simulink model "Neurofeedback_StateSpace_Neurodynamics"  (R2021b)
settings: Solver=VariableStepAuto  StartTime=0.0  StopTime=300  FixedStep=0.1  RelTol=1e-3
settings Model: Creator=mdls3  LastModifiedBy=mariodelossantos

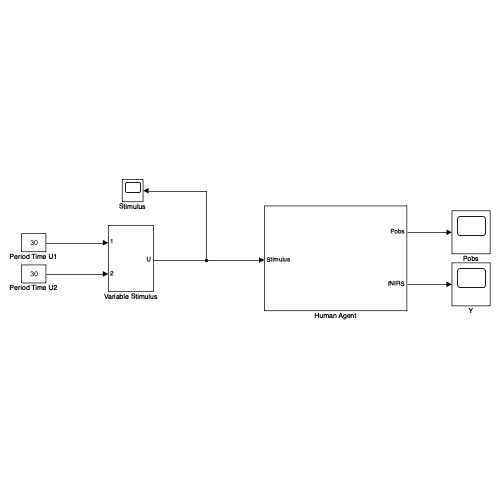
[thumbnail: Simulink's stored preview of the top-level diagram]
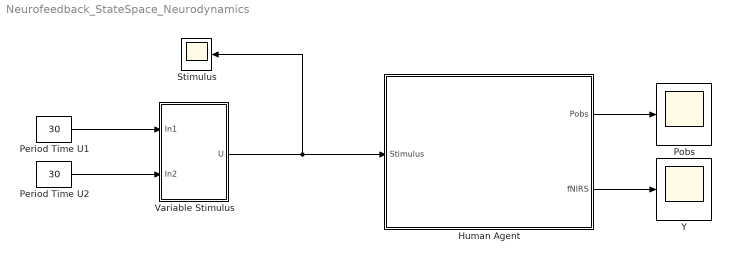
== system Neurofeedback_StateSpace_Neurodynamics ==
  Human Agent : Subsystem
  Period Time U1 : Constant  Value=30
  Period Time U2 : Constant  Value=30
  Pobs : Scope
  Stimulus : Scope
  Variable Stimulus : Subsystem
  Y : Scope
  wires:
  Period Time U1/1 -> Variable Stimulus/1(In1)
  Period Time U2/1 -> Variable Stimulus/2(In2)
  Variable Stimulus/1(U) -> Stimulus/1, Human Agent/1(Stimulus)
  Human Agent/2(fNIRS) -> Y/1
  Human Agent/1(Pobs) -> Pobs/1

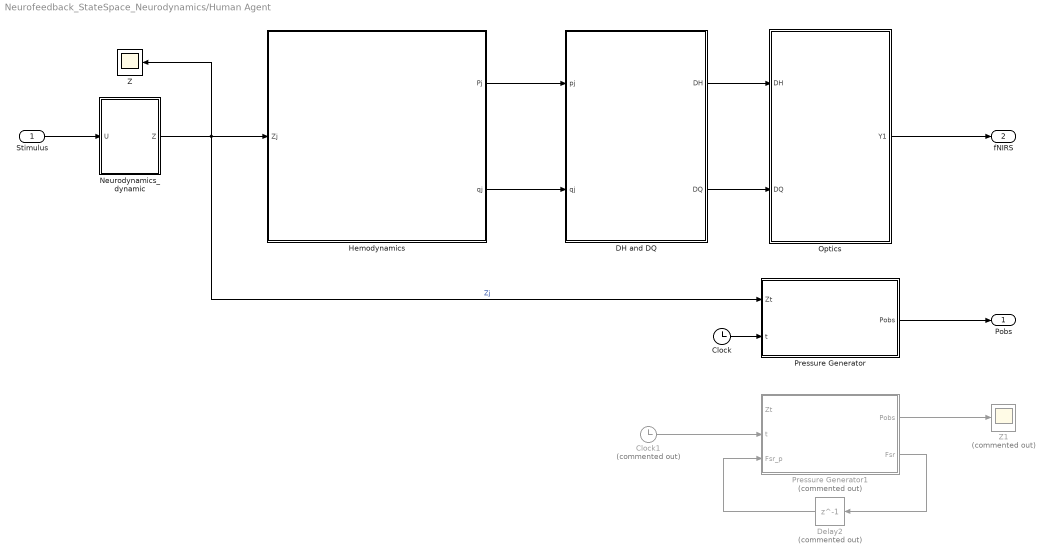
== system Neurofeedback_StateSpace_Neurodynamics/Human Agent ==
  Stimulus : Inport
  Clock : Clock
  Clock1 : Clock  Commented=on
  DH and DQ : Subsystem
  Delay2 : Delay  Commented=on  DelayLength=1  InitialCondition=0.0001
  Hemodynamics : Subsystem
  Neurodynamics_dynamic : Subsystem
  Optics : Subsystem
  Pressure Generator : MATLAB Function  TreatAsAtomicUnit=on
  Pressure Generator1 : MATLAB Function  Commented=on  TreatAsAtomicUnit=on
  Z : Scope
  Z1 : Scope  Commented=on
  Pobs : Outport
  fNIRS : Outport  Port=2
  wires:
  Hemodynamics/1(Pj) -> DH and DQ/1(pj)
  Hemodynamics/2(qj) -> DH and DQ/2(qj)
  Neurodynamics_dynamic/1(Z) -> Pressure Generator/1(Zt), Z/1, Hemodynamics/1(Zj)  "Zj"
  Stimulus/1 -> Neurodynamics_dynamic/1(U)
  DH and DQ/1(DH) -> Optics/1(DH)
  DH and DQ/2(DQ) -> Optics/2(DQ)
  Optics/1(Y1) -> fNIRS/1
  Clock/1 -> Pressure Generator/2(t)
  Pressure Generator/1(Pobs) -> Pobs/1
  Delay2/1 -> Pressure Generator1/3(Fsr_p)
  Pressure Generator1/1(Pobs) -> Z1/1
  Clock1/1 -> Pressure Generator1/2(t)
  Pressure Generator1/2(Fsr) -> Delay2/1

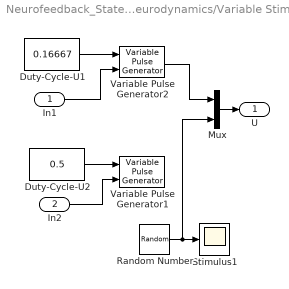
== system Neurofeedback_StateSpace_Neurodynamics/Variable Stimulus ==
  In1 : Inport
  In2 : Inport  Port=2
  Duty-Cycle-U1 : Constant  Value=0.16667  OutMin=[0]  OutMax=[0.8]
  Duty-Cycle-U2 : Constant  Value=0.5  OutMin=[0]  OutMax=[0.8]
  Mux : Mux  Inputs=2
  Random Number : RandomNumber  Variance=0.1  SampleTime=0.03
  Stimulus1 : Scope
  Variable Pulse Generator1 : VariablePulseGenerator  RunAtFixedTimeIntervals=on  SampleTime=1/10.4
  Variable Pulse Generator2 : VariablePulseGenerator  RunAtFixedTimeIntervals=on  SampleTime=1/10.4
  U : Outport
  wires:
  In2/1 -> Variable Pulse Generator1/2
  Mux/1 -> U/1
  Duty-Cycle-U2/1 -> Variable Pulse Generator1/1
  In1/1 -> Variable Pulse Generator2/2
  Duty-Cycle-U1/1 -> Variable Pulse Generator2/1
  Variable Pulse Generator2/1 -> Mux/1
  Random Number/1 -> Mux/2, Stimulus1/1

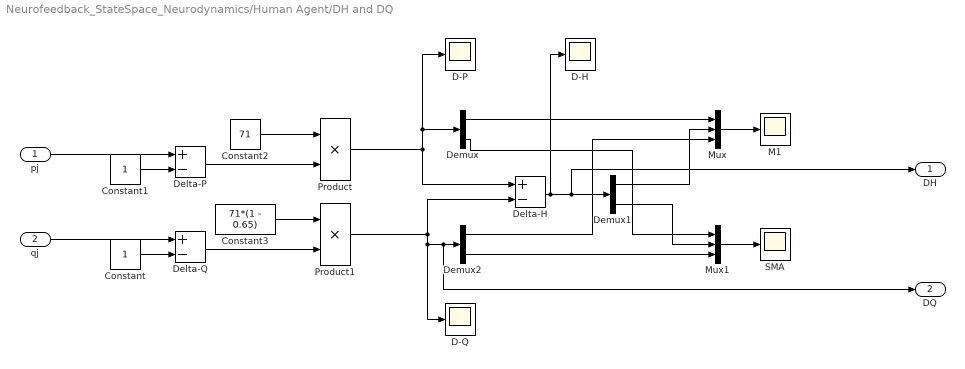
== system Neurofeedback_StateSpace_Neurodynamics/Human Agent/DH and DQ ==
  pj : Inport
  qj : Inport  Port=2
  Constant : Constant
  Constant1 : Constant
  Constant2 : Constant  Value=71
  Constant3 : Constant  Value=71*(1 - 0.65)
  D-H : Scope
  D-P : Scope
  D-Q : Scope
  Delta-H : Sum  Inputs=+-
  Delta-P : Sum  Inputs=+-
  Delta-Q : Sum  Inputs=+-
  Demux : Demux  Outputs=2
  Demux1 : Demux  Outputs=2
  Demux2 : Demux  Outputs=2
  M1 : Scope
  Mux : Mux  Inputs=3
  Mux1 : Mux  Inputs=3
  Product : Product
  Product1 : Product
  SMA : Scope
  DH : Outport
  DQ : Outport  Port=2
  wires:
  Constant2/1 -> Product/1
  Delta-Q/1 -> Product1/2
  Constant3/1 -> Product1/1
  Demux2/2 -> Mux1/3
  pj/1 -> Delta-P/1
  Mux1/1 -> SMA/1
  Demux/2 -> Mux1/1
  Mux/1 -> M1/1
  Constant/1 -> Delta-Q/2
  Delta-P/1 -> Product/2
  Product1/1 -> DQ/1, Demux2/1, D-Q/1, Delta-H/2
  qj/1 -> Delta-Q/1
  Demux/1 -> Mux/1
  Delta-H/1 -> DH/1, Demux1/1, D-H/1
  Demux1/1 -> Mux/2
  Demux1/2 -> Mux1/2
  Product/1 -> Demux/1, D-P/1, Delta-H/1
  Demux2/1 -> Mux/3
  Constant1/1 -> Delta-P/2

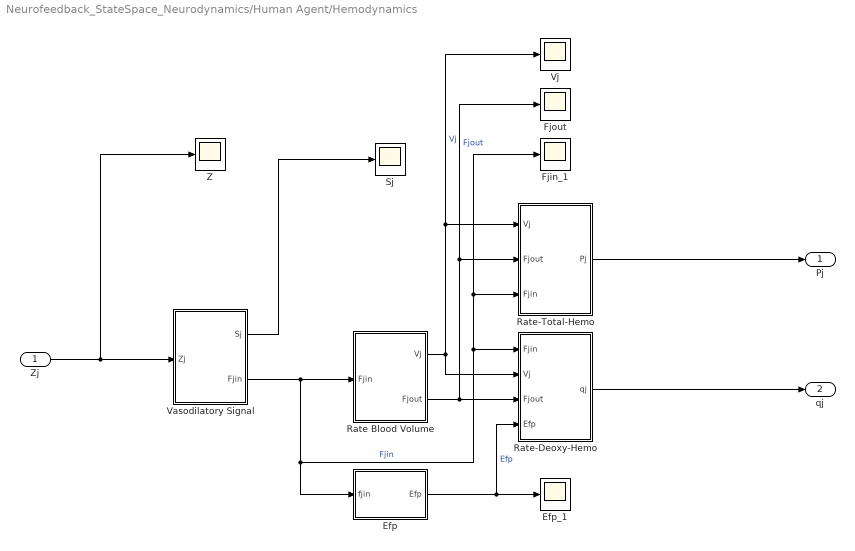
== system Neurofeedback_StateSpace_Neurodynamics/Human Agent/Hemodynamics ==
  Zj : Inport
  Efp : MATLAB Function  TreatAsAtomicUnit=on
  Efp_1 : Scope
  Fjin_1 : Scope
  Fjout : Scope
  Rate Blood Volume : Subsystem
  Rate-Deoxy-Hemo : Subsystem
  Rate-Total-Hemo : Subsystem
  Sj : Scope
  Vasodilatory Signal : Subsystem
  Vj : Scope
  Z : Scope
  Pj : Outport
  qj : Outport  Port=2
  wires:
  Rate-Deoxy-Hemo/1(qj) -> qj/1
  Zj/1 -> Vasodilatory Signal/1(Zj), Z/1
  Vasodilatory Signal/1(Sj) -> Sj/1
  Rate Blood Volume/2(Fjout) -> Fjout/1, Rate-Total-Hemo/2(Fjout), Rate-Deoxy-Hemo/3(Fjout)  "Fjout"
  Rate Blood Volume/1(Vj) -> Vj/1, Rate-Total-Hemo/1(Vj), Rate-Deoxy-Hemo/2(Vj)  "Vj"
  Rate-Total-Hemo/1(Pj) -> Pj/1
  Efp/1(Efp) -> Rate-Deoxy-Hemo/4(Efp), Efp_1/1  "Efp"
  Vasodilatory Signal/2(Fjin) -> Efp/1(fjin), Fjin_1/1, Rate-Total-Hemo/3(Fjin), Rate-Deoxy-Hemo/1(Fjin), Rate Blood Volume/1(Fjin)  "Fjin"

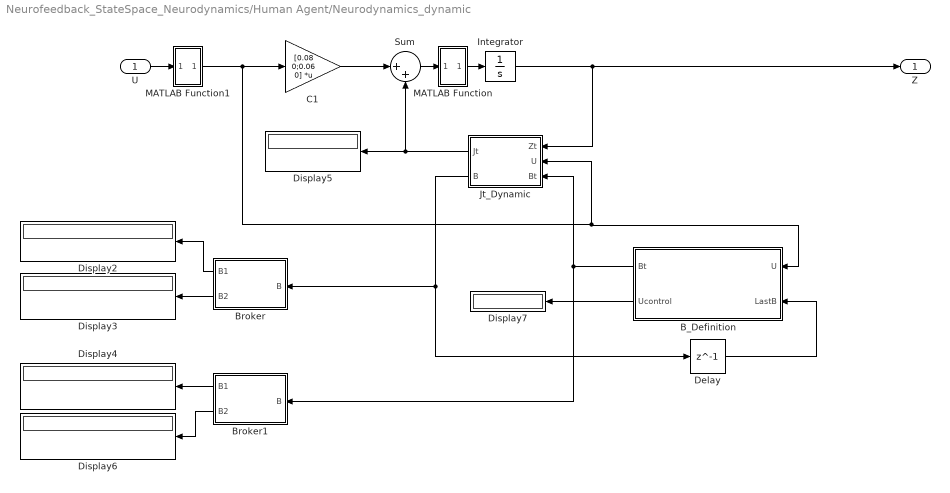
== system Neurofeedback_StateSpace_Neurodynamics/Human Agent/Neurodynamics_dynamic ==
  U : Inport
  B_Definition : MATLAB Function  TreatAsAtomicUnit=on
  Broker : MATLAB Function  TreatAsAtomicUnit=on
  Broker1 : MATLAB Function  TreatAsAtomicUnit=on
  C1 : Gain  Gain=[0.08 0;0.06 0]  Multiplication=Matrix(K*u) (u vector)
  Delay : Delay  DelayLength=1  InitialCondition=0
  Display{2..7} (6 alike) : Display
  Integrator : Integrator
  Jt_Dynamic : MATLAB Function  TreatAsAtomicUnit=on
  MATLAB Function : MATLAB Function  TreatAsAtomicUnit=on
  MATLAB Function1 : MATLAB Function  TreatAsAtomicUnit=on
  Sum : Sum  Inputs=|++
  Z : Outport
  wires:
  Integrator/1 -> Z/1, Jt_Dynamic/1(Zt)
  C1/1 -> Sum/1
  U/1 -> MATLAB Function1/1(Z)
  Sum/1 -> MATLAB Function/1(Z)
  MATLAB Function1/1(Zn) -> C1/1, B_Definition/1(U), Jt_Dynamic/2(U)
  MATLAB Function/1(Zn) -> Integrator/1
  Jt_Dynamic/1(Jt) -> Display5/1, Sum/2
  Delay/1 -> B_Definition/2(LastB)
  Jt_Dynamic/2(B) -> Broker/1(B), Delay/1
  Broker/1(B1) -> Display2/1
  Broker/2(B2) -> Display3/1
  B_Definition/1(Bt) -> Jt_Dynamic/3(Bt), Broker1/1(B)
  Broker1/2(B2) -> Display6/1
  Broker1/1(B1) -> Display4/1
  B_Definition/2(Ucontrol) -> Display7/1

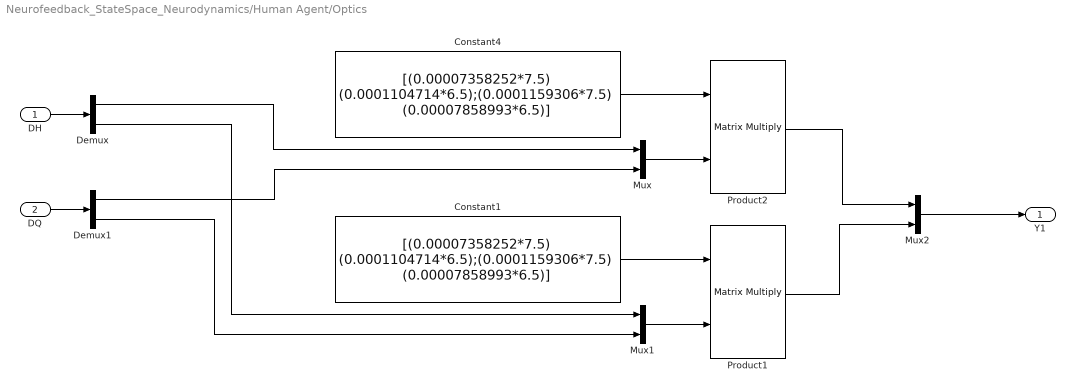
== system Neurofeedback_StateSpace_Neurodynamics/Human Agent/Optics ==
  DH : Inport
  DQ : Inport  Port=2
  Constant1 : Constant  Value=[(0.00007358252*7.5) (0.0001104714*6.5);(0.0001159306*7.5) (0.00007858993*6.5)]
  Constant4 : Constant  Value=[(0.00007358252*7.5) (0.0001104714*6.5);(0.0001159306*7.5) (0.00007858993*6.5)]
  Demux : Demux  Outputs=2
  Demux1 : Demux  Outputs=2
  Mux : Mux  Inputs=2
  Mux1 : Mux  Inputs=2
  Mux2 : Mux  Inputs=2
  Product1 : Product  Multiplication=Matrix(*)
  Product2 : Product  Multiplication=Matrix(*)
  Y1 : Outport
  wires:
  Mux/1 -> Product2/2
  Product2/1 -> Mux2/1
  Mux1/1 -> Product1/2
  Product1/1 -> Mux2/2
  Constant1/1 -> Product1/1
  DH/1 -> Demux/1
  Demux/1 -> Mux/1
  Demux/2 -> Mux1/1
  DQ/1 -> Demux1/1
  Constant4/1 -> Product2/1
  Demux1/1 -> Mux/2
  Demux1/2 -> Mux1/2
  Mux2/1 -> Y1/1

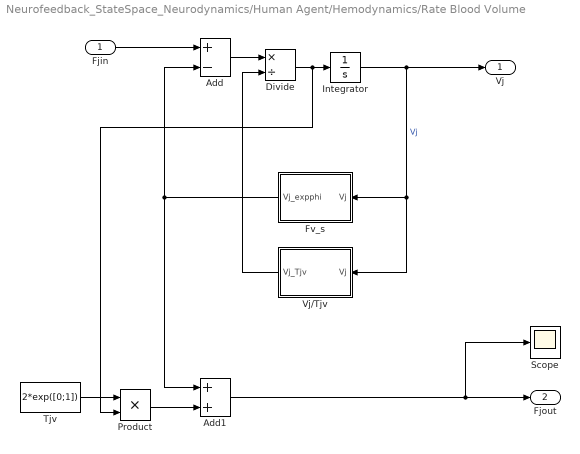
== system Neurofeedback_StateSpace_Neurodynamics/Human Agent/Hemodynamics/Rate Blood Volume ==
  Fjin : Inport
  Add : Sum  Inputs=+-
  Add1 : Sum
  Divide : Product  Inputs=*/
  Fv_s : MATLAB Function  TreatAsAtomicUnit=on
  Integrator : Integrator  InitialCondition=exp([0;0])
  Product : Product
  Scope : Scope
  Tjv : Constant  Value=2*exp([0;1])
  Vj/Tjv : MATLAB Function  TreatAsAtomicUnit=on
  Vj : Outport
  Fjout : Outport  Port=2
  wires:
  Fjin/1 -> Add/1
  Integrator/1 -> Vj/1, Vj/Tjv/1(Vj), Fv_s/1(Vj)  "Vj"
  Divide/1 -> Product/2, Integrator/1
  Fv_s/1(Vj_expphi) -> Add/2, Add1/1
  Add/1 -> Divide/1
  Vj/Tjv/1(Vj_Tjv) -> Divide/2
  Product/1 -> Add1/2
  Tjv/1 -> Product/1
  Add1/1 -> Scope/1, Fjout/1

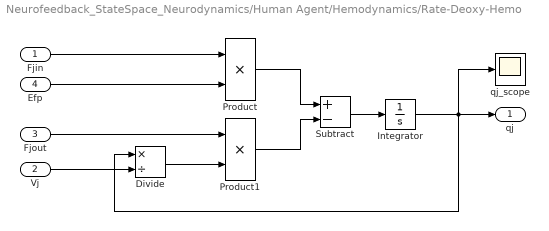
== system Neurofeedback_StateSpace_Neurodynamics/Human Agent/Hemodynamics/Rate-Deoxy-Hemo ==
  Fjin : Inport
  Vj : Inport  Port=2
  Fjout : Inport  Port=3
  Efp : Inport  Port=4
  Divide : Product  Inputs=*/
  Integrator : Integrator  InitialCondition=exp([0;0])
  Product : Product
  Product1 : Product
  Subtract : Sum  Inputs=+-
  qj_scope : Scope
  qj : Outport
  wires:
  Efp/1 -> Product/2
  Divide/1 -> Product1/2
  Subtract/1 -> Integrator/1
  Integrator/1 -> qj/1, Divide/1, qj_scope/1
  Vj/1 -> Divide/2
  Product1/1 -> Subtract/2
  Fjin/1 -> Product/1
  Fjout/1 -> Product1/1
  Product/1 -> Subtract/1

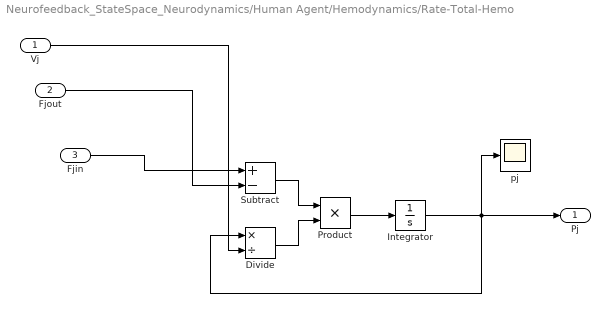
== system Neurofeedback_StateSpace_Neurodynamics/Human Agent/Hemodynamics/Rate-Total-Hemo ==
  Vj : Inport
  Fjout : Inport  Port=2
  Fjin : Inport  Port=3
  Divide : Product  Inputs=*/
  Integrator : Integrator  InitialCondition=exp([0;0])
  Product : Product
  Subtract : Sum  Inputs=+-
  pj : Scope
  Pj : Outport
  wires:
  Fjout/1 -> Subtract/2
  Product/1 -> Integrator/1
  Vj/1 -> Divide/2
  Subtract/1 -> Product/1
  Fjin/1 -> Subtract/1
  Divide/1 -> Product/2
  Integrator/1 -> Pj/1, pj/1, Divide/1

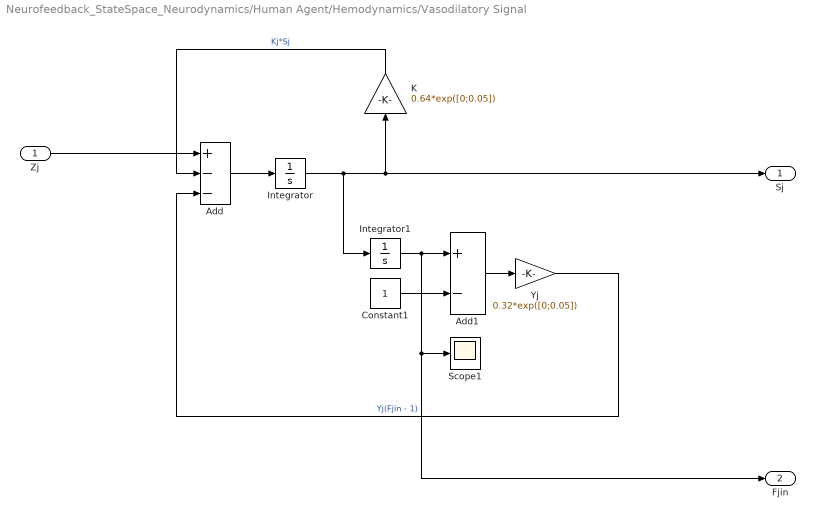
== system Neurofeedback_StateSpace_Neurodynamics/Human Agent/Hemodynamics/Vasodilatory Signal ==
  Zj : Inport
  Add : Sum  Inputs=+--
  Add1 : Sum  Inputs=+-
  Constant1 : Constant
  Integrator : Integrator
  Integrator1 : Integrator  InitialCondition=exp([0;0])
  K : Gain  Gain=0.64*exp([0;0.05])
  Scope1 : Scope
  Yj : Gain  Gain=0.32*exp([0;0.05])
  Sj : Outport
  Fjin : Outport  Port=2
  wires:
  Add1/1 -> Yj/1
  K/1 -> Add/2  "Kj*Sj"
  Constant1/1 -> Add1/2
  Zj/1 -> Add/1
  Integrator1/1 -> Fjin/1, Scope1/1, Add1/1
  Integrator/1 -> Sj/1, K/1, Integrator1/1
  Add/1 -> Integrator/1
  Yj/1 -> Add/3  "Yj(Fjin - 1)"

== matlab function Neurofeedback_StateSpace_Neurodynamics/Human Agent/Hemodynamics/Efp ==
  data: fjin input; Efp output
function Efp= fcn(fjin)

Efp = (1 - (1 - 0.32).^ (1 ./ fjin))/0.32;

== matlab function Neurofeedback_StateSpace_Neurodynamics/Human Agent/Pressure Generator ==
  data: Zt input; Pobs output; t input
function Pobs = fcn(Zt, t)
    R=28.2; %Resistor [Ohms];
    C=1.7; %Capacitor [Faradays];
    V= Zt(1); %Voltage or system reference;
    Vc = V * (exp(-t/(R*C))); % Voltage at the capacitor  
    
Pobs = Vc;

== matlab function Neurofeedback_StateSpace_Neurodynamics/Human Agent/Pressure Generator1 ==
  data: Zt input; Pobs output; t input; Fsr_p input; Fsr output
function [Pobs,Fsr] = PressureGenerator_sensor(Zt, t,Fsr_p)
    C = 2.5; % 0.1F
    Vcc = 500; %Considering 5V as a real sensor, the value is on mV
    Rf = 1000; %Fixed resistor 10k ohms
    kgf = 0.1019716213; % 1N = 0.1019716213 kgf
    Fsr = 0;
    Fsrforce = 0;

    Vout = Zt(1) * (1 - exp( -t / C)); %Emulation of the capacitor
    Fsr = (Vcc - Vout * Rf) / Vout;
    FsConductance = 1000000; %Sensor conductance in uOhms
    FsConductance = FsConductance / Fsr;
    if FsConductance <= 1000
        Fsrforce = FsConductance / 80; %Force on Newtons
    else
        Fsrforce = FsConductance - 1000;
        Fsrforce = Fsrforce / 30;
    end
    
Pobs = Fsrforce;

end

== matlab function Neurofeedback_StateSpace_Neurodynamics/Human Agent/Hemodynamics/Rate Blood Volume/Fv_s ==
  data: Vj input; Vj_expphi output
function Vj_expphi = fcn(Vj)
phi = 0.32;
Vj_expphi = Vj.^(1/phi);

== matlab function Neurofeedback_StateSpace_Neurodynamics/Human Agent/Hemodynamics/Rate Blood Volume/Vj//Tjv ==
  data: Vj input; Vj_Tjv output
function Vj_Tjv = fcn(Vj)
    Tjv = 2*exp([0;1]);
    Tj = 2*exp([0;0.05]);
Vj_Tjv =(Tj.*Tjv.*Vj);

== matlab function Neurofeedback_StateSpace_Neurodynamics/Human Agent/Neurodynamics_dynamic/B_Definition ==
  settings: updateMethod=DISCRETE
  data: U input; Bt output; LastB input; Ucontrol output
function [Bt, Ucontrol] = B_Definition(U, LastB)
   Bt = zeros(2, 2, 2);
   %Control extraction and weight
   Ucontrol = U(2) * (0.2 + rand(1) * (1-0.2));
   Threshold = 0.2;
    if(Ucontrol < Threshold) %Random Ucontrol to test
        min = -1; 
        max = 1.5;
        n = 2;
        r1 = min + rand(n)*(max-min);
        r2 = min + rand(n)*(max-min);
        %Bt(:,:,1) = r1(:,:);
        Bt(:,:,2) = r2(:,:);
    else
       Bt = LastB;
    end

== matlab function Neurofeedback_StateSpace_Neurodynamics/Human Agent/Neurodynamics_dynamic/Broker ==
  data: B input; B1 output; B2 output
function [B1, B2] = fcn(B)
B1 = B(:,:,1);
B2 = B(:,:,2);

== matlab function Neurofeedback_StateSpace_Neurodynamics/Human Agent/Neurodynamics_dynamic/Broker1 ==
  data: B input; B1 output; B2 output
function [B1, B2] = fcn(B)
B1 = B(:,:,1);
B2 = B(:,:,2);

== matlab function Neurofeedback_StateSpace_Neurodynamics/Human Agent/Neurodynamics_dynamic/Jt_Dynamic ==
  data: Zt input; U input; Jt output; Bt input; B output
function [Jt, B] = fcn(Zt, U, Bt)

   A = [-0.16 -0.49;-0.02 -0.33];
   nRegions  = size(A,1);

   B = zeros(2,2,2);
   a = 0;
   B1 = [0 0; 0 0]; %There must be a B per stimulus
   B2 = [-0.02 -0.77; 0.33 -1.31];

   if Bt(:,:,2) ~= B(:,:,2)
       B(:,:,:) = Bt(:,:,:);
   else
          B(:,:,1) = B1;
          B(:,:,2) = B2;
   end
   M = size(U,1); %nStimuli
   assert(M == size(B,3),...
        'Unexpected number of induced connectivity parameters B.');

    simulationLength = size(U,2);
    for t = 1:simulationLength
       T = zeros(nRegions); %nRegions x nRegions
                   for uu = 1:M % Sum (Uj * Bj)
                       tmp = U(uu,t) * B(:,:,uu);
                       T = -0.5 * exp(T + tmp);  
                   end
            SI = diag(A);
    end
        A =  A - diag(exp(SI) + (SI));
Jt = (A*Zt) + (T*Zt);

== matlab function Neurofeedback_StateSpace_Neurodynamics/Human Agent/Neurodynamics_dynamic/MATLAB Function ==
  data: Z input; Zn output
function Zn = fcn(Z)

Zn = Z(:,1);

== matlab function Neurofeedback_StateSpace_Neurodynamics/Human Agent/Neurodynamics_dynamic/MATLAB Function1 ==
  data: Z input; Zn output
function Zn = fcn(Z)

Zn = Z(:,1);
